simulink model "Closed_loop"  (R2021a)
settings: Solver=FixedStepAuto  StartTime=0.0  StopTime=inf  RelTol=1e-3
InitFcn:
  | clear all;
  | s = serialport('COM3', 115200);
  | write(s, [251 0], 'uint8');
  | clear s;
StopFcn:
  | clear s;
libraries: pid_lib x1, aerolibanimutils x1
settings Model: Creator=PSVN_Controls2  LastModifiedBy=SHRENI MALYALA
settings SolverCC: AlgebraicLoopSolver=TrustRegion
settings DebuggingCC: SFMachineParentedDataDiag=warning

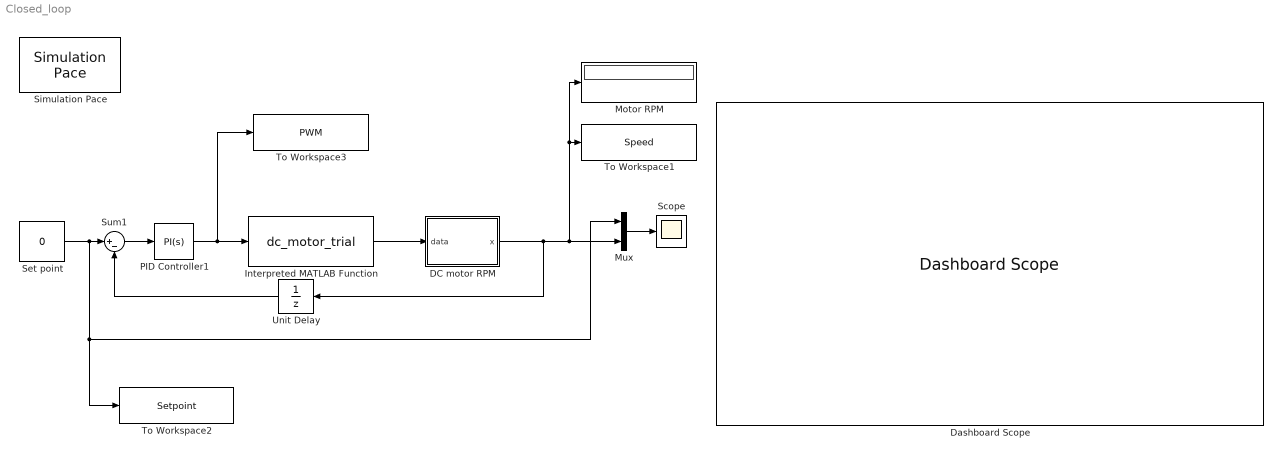
== system Closed_loop ==
  "DC motor RPM " : MATLAB Function  TreatAsAtomicUnit=on
  Dashboard Scope : DashboardScope  Ymin=0  Ymax=4000
  Interpreted MATLAB Function : MATLABFcn  MATLABFcn=dc_motor_trial  OutputDimensions=[1,2]  Output1D=off
  Motor RPM : Display
  Mux : Mux  Inputs=2
  PID Controller1 : pid_lib/PID Controller  Controller=PI  Form=Ideal  TimeDomain=Continuous-time  UseExternalTs=off  SampleTime=0.015  IntegratorMethod=Forward Euler  FilterMethod=Forward Euler  ControllerParametersSource=internal  P=0.0177  I=4.62  D=0  UseFilter=on  N=100  TunerSelectOption=Transfer Function Based (PID Tuner App)  InitialConditionSource=internal  InitialConditionForIntegrator=0  InitialConditionForFilter=0  DifferentiatorICPrevScaledInput=0  ExternalReset=none  TrackingMode=off  Kt=1  LimitOutput=on  SatLimitsSource=internal  UpperSaturationLimit=255  LowerSaturationLimit=0  LinearizeAsGain=on  AntiWindupMode=none  Kb=1  POutMin=[]  POutMax=[]  IOutMin=[]  IOutMax=[]  DOutMin=[]  DOutMax=[]  NOutMin=[]  NOutMax=[]  SumOutMin=[]  SumOutMax=[]  SaturationOutMin=[]  SaturationOutMax=[]  PParamMin=[]  PParamMax=[]  IParamMin=[]  IParamMax=[]  DParamMin=[]  DParamMax=[]  NParamMin=[]  NParamMax=[]  KbParamMin=[]  KbParamMax=[]  KtParamMin=[]  KtParamMax=[]  KbOutMin=[]  KbOutMax=[]  KtOutMin=[]  KtOutMax=[]  IntegratorOutMin=[]  IntegratorOutMax=[]  FilterOutMin=[]  FilterOutMax=[]  SumI1OutMin=[]  SumI1OutMax=[]  SumI2OutMin=[]  SumI2OutMax=[]  SumI3OutMin=[]  SumI3OutMax=[]  SumI4OutMin=[]  SumI4OutMax=[]  SumDOutMin=[]  SumDOutMax=[]  DifferentiatorOutMin=[]  DifferentiatorOutMax=[]  FilterDiffOutCoefMin=[]  FilterDiffOutCoefMax=[]  ReciprocalOutMin=[]  ReciprocalOutMax=[]  SumDenOutMin=[]  SumDenOutMax=[]  SumNumOutMin=[]  SumNumOutMax=[]  DivideOutMin=[]  DivideOutMax=[]  UdiffTsProdOutMin=[]  UdiffTsProdOutMax=[]  NTsProdOutMin=[]  NTsProdOutMax=[]  UintegralTsProdOutMin=[]  UintegralTsProdOutMax=[]  UngainTsProdOutMin=[]  UngainTsProdOutMax=[]  IntegratorContinuousStateAttributes=''  IntegratorStateMustResolveToSignalObject=off  IntegratorRTWStateStorageClass=Auto  FilterContinuousStateAttributes=''  FilterStateMustResolveToSignalObject=off  FilterRTWStateStorageClass=Auto  ParallelPVariant=Passthrough  IdealPVariant=InternalParameters  IVariant=InternalParameters  DVariant=Disabled  IntegratorVariant=Continuous  SatVariant=Enabled  AWVariant=Passthrough  PCopyVariant=Disabled  TRVariant=Disabled  FdbkBlocksVariant=Forward  IdealPFdbkVariant=Disabled  SatFdbkVariant=Disabled  DerivativeFilterVariant=Disabled  NVariant=Disabled  NCopyVariant=Disabled_SignalSpec  FilterICVariant=Disabled  IntegratorICVariant=InternalICs  ExternalResetVariant=Disabled  TRSumVariant=Passthrough  SumFdbkVariant=Disabled  SumVariant=Sum_PI  TsampFilterVariant=InternalTs  TsampNgainVariant=Passthrough  TsampIntegralVariant=Passthrough  ExternalSaturationOutDataTypeStr=Inherit: Same as second input
  Scope : Scope
  Set point : Constant  Value=0  SampleTime=0.015
  Simulation Pace : aerolibanimutils/Simulation Pace  SimulationPace=1  SleepMode=MATLAB Thread  OutputPaceError=off  SampleTime=0.015
  Sum1 : Sum  Inputs=|+-
  To Workspace1 : ToWorkspace  VariableName=Speed  SaveFormat=Timeseries  SampleTime=0.015
  To Workspace2 : ToWorkspace  VariableName=Setpoint  SaveFormat=Timeseries  SampleTime=0.015
  To Workspace3 : ToWorkspace  VariableName=PWM  SaveFormat=Timeseries  SampleTime=0.015
  Unit Delay : UnitDelay  SampleTime=0.015  HasFrameUpgradeWarning=on
  wires:
  Interpreted MATLAB Function/1 -> "DC motor RPM "/1(data)
  "DC motor RPM "/1(x) -> To Workspace1/1, Motor RPM/1, Mux/2, Unit Delay/1
  Sum1/1 -> PID Controller1/1
  PID Controller1/1 -> To Workspace3/1, Interpreted MATLAB Function/1
  Set point/1 -> To Workspace2/1, Mux/1, Sum1/1
  Unit Delay/1 -> Sum1/2
  Mux/1 -> Scope/1

== matlab function Closed_loop/DC motor RPM  ==
  data: data input; x output
function x  = PWM(data)

F = data(:,1)*256;
r = data(:,2);
x = (F+r)*8.982025;

end
